simulink model "Estimation_Kphi_experiment"  (R2022b)
settings: Solver=FixedStepAuto  StartTime=0.0  StopTime=50  RelTol=1e-3  EnableMultiTasking=on
libraries: arduinolib x4
settings Model: SimulationMode=external  ExtModeTrigDuration=2  Creator=gotta  LastModifiedBy=gotta
settings OptimizationCC: EnhancedBackFolding=on  PassReuseOutputArgsAs=Individual arguments  ZeroExternalMemoryAtStartup=off  ZeroInternalMemoryAtStartup=off  MaxStackSize=64  OptimizeBlockOrder=speed  DifferentSizesBufferReuse=on  OptimizationCustomize=off  EfficientTunableParamExpr=on
settings DebuggingCC: ParameterTunabilityLossMsg=error
settings HardwareCC: ProdBitPerPointer=32  ProdBitPerSizeT=32  ProdBitPerPtrDiffT=32  ProdLargestAtomicInteger=Long  ProdLargestAtomicFloat=Double  ProdWordSize=32  ProdHWDeviceType=ARM Compatible->ARM Cortex
settings SFSimCC: MATLABDynamicMemAlloc=off
settings RTWCC: Description=Embedded Coder  SystemTargetFile=ert.tlc  HardwareBoard=ESP32-WROOM(Arduino Compatible)  TLCOptions="-aInlineSetEventsForThisBaseRateFcn=TLC_FALSE -aSuppressMultiTaskScheduler=TLC_FALSE  -aRateBasedStepFcn=0"  TemplateMakefile=ert_default_tmf  Toolchain=ESP32  BuildConfiguration=Faster Runs
settings CodeAppCC: ForceParamTrailComments=on  IgnoreCustomStorageClasses=off  OperatorAnnotations=on  SimulinkDataObjDesc=on  SFDataObjDesc=on  InsertBlockDesc=on
settings ERTTargetCC: SupportContinuousTime=on  SupportVariableSizeSignals=on  ExtModeTransport=3  ExtModeStaticAlloc=on  ExtModeAutomaticAllocSize=off  ExtModeStaticAllocSize=65536  ExtModeMexFile=ext_xcp  ExtModeIntrfLevel=Level2 - Open

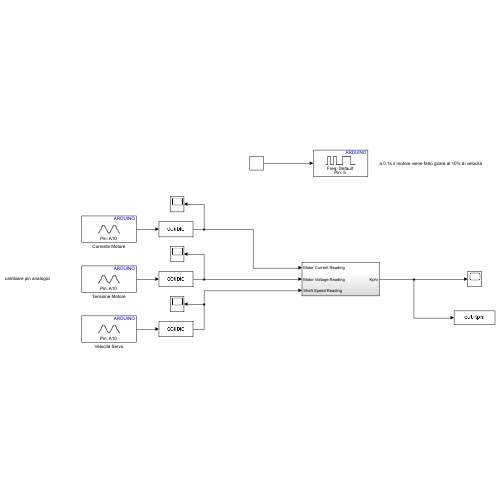
[thumbnail: Simulink's stored preview of the top-level diagram]
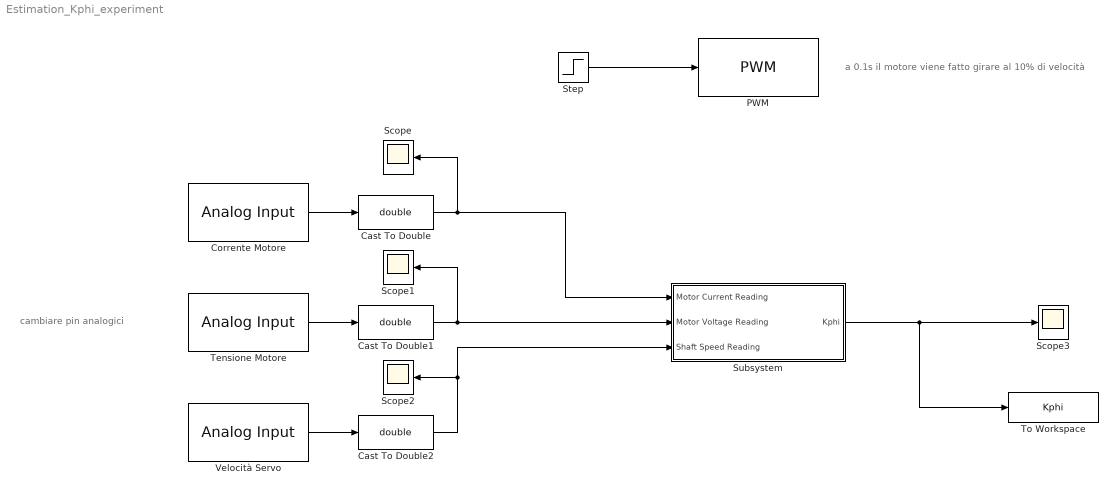
== system Estimation_Kphi_experiment ==
  note: cambiare pin analogici
  note: a 0.1s il motore viene fatto girare al 10% di velocità
  Cast To Double : DataTypeConversion  OutDataTypeStr=double  SaturateOnIntegerOverflow=off  RndMeth=Floor
  Cast To Double1 : DataTypeConversion  OutDataTypeStr=double  SaturateOnIntegerOverflow=off  RndMeth=Floor
  Cast To Double2 : DataTypeConversion  OutDataTypeStr=double  SaturateOnIntegerOverflow=off  RndMeth=Floor
  Corrente Motore : arduinolib/Analog Input  pinNumber=10  ReadResultsOnly=off  ConversionTriggerSource=Software  ExternalTriggerType=uint32( 0 )  OutputDataType=uint16  EnableConversionCompleteNotify=off  EnableOuputStatus=off  SampleTime=0.001  blockPlatform=arduino
  PWM : arduinolib/PWM  pinNumber=5  frequencyType=Default  desiredFrequency=490.2  achievableFrequency=490.2
  Scope{,1..3} (4 alike) : Scope
  Step : Step  Time=0.1  After=0.1  SampleTime=0
  Subsystem : Subsystem
  Tensione Motore : arduinolib/Analog Input  pinNumber=10  ReadResultsOnly=off  ConversionTriggerSource=Software  ExternalTriggerType=uint32( 0 )  OutputDataType=uint16  EnableConversionCompleteNotify=off  EnableOuputStatus=off  SampleTime=0.001  blockPlatform=arduino
  To Workspace : ToWorkspace  VariableName=Kphi  SaveFormat=Timeseries  SampleTime=-1
  Velocità Servo : arduinolib/Analog Input  pinNumber=10  ReadResultsOnly=off  ConversionTriggerSource=Software  ExternalTriggerType=uint32( 0 )  OutputDataType=uint16  EnableConversionCompleteNotify=off  EnableOuputStatus=off  SampleTime=0.001  blockPlatform=arduino
  wires:
  Corrente Motore/1 -> Cast To Double/1
  Cast To Double/1 -> Subsystem/1(Motor Current Reading), Scope/1
  Step/1 -> PWM/1
  Velocità Servo/1 -> Cast To Double2/1
  Tensione Motore/1 -> Cast To Double1/1
  Cast To Double1/1 -> Scope1/1, Subsystem/2(Motor Voltage Reading)
  Cast To Double2/1 -> Subsystem/3(Shaft Speed Reading), Scope2/1
  Subsystem/1(Kphi) -> To Workspace/1, Scope3/1

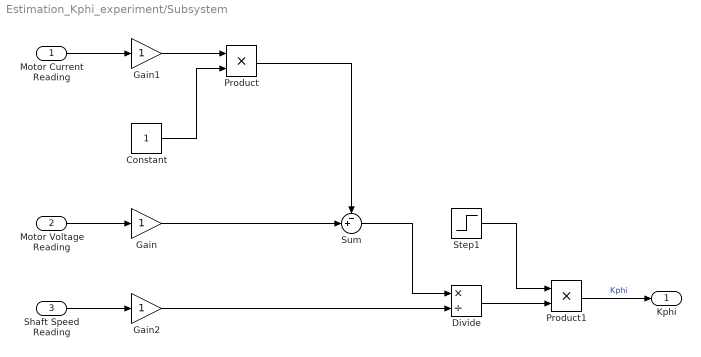
== system Estimation_Kphi_experiment/Subsystem ==
  Motor Current Reading : Inport
  Motor Voltage Reading : Inport  Port=2
  Shaft Speed Reading : Inport  Port=3
  Constant : Constant
  Divide : Product  Inputs=*/
  Gain : Gain
  Gain1 : Gain
  Gain2 : Gain
  Product : Product
  Product1 : Product
  Step1 : Step  Time=0.25  SampleTime=0
  Sum : Sum  Inputs=-+|
  Kphi : Outport
  wires:
  Product1/1 -> Kphi/1  "Kphi"
  Divide/1 -> Product1/2
  Step1/1 -> Product1/1
  Gain/1 -> Sum/2
  Product/1 -> Sum/1
  Gain2/1 -> Divide/2
  Constant/1 -> Product/2
  Gain1/1 -> Product/1
  Sum/1 -> Divide/1
  Motor Current Reading/1 -> Gain1/1
  Motor Voltage Reading/1 -> Gain/1
  Shaft Speed Reading/1 -> Gain2/1
